simulink model "Test_Arithmetic_Operation_Word_Comparator_Equal"  (Simulink 8.7)
settings: Solver=ode45  StartTime=0.0  StopTime=len  RelTol=1e-3
libraries: Miscellaneous x2, Arithmetic_Operations_Lib x1
settings Model: Creator=uzivatel  LastModifiedBy=Jozko Mrkvicka
settings DebuggingCC: SolverPrmCheckMsg=warning  StateNameClashWarn=warning

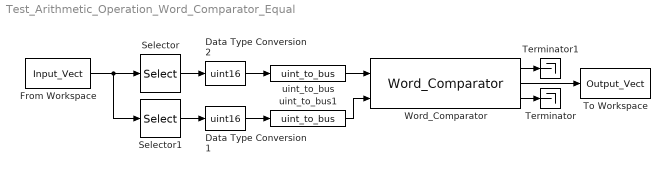
== system Test_Arithmetic_Operation_Word_Comparator_Equal ==
  Data Type Conversion1 : DataTypeConversion  OutDataTypeStr=uint16
  Data Type Conversion2 : DataTypeConversion  OutDataTypeStr=uint16
  From Workspace : FromWorkspace  VariableName=Input_Vect  SampleTime=1  Interpolate=off  OutputAfterFinalValue=Holding final value
  Selector : Selector  IndexMode=Zero-based  InputPortWidth=2  SampleTime=1  IndexOptions=Index vector (dialog)  Indices=0  OutputSizes=1
  Selector1 : Selector  IndexMode=Zero-based  InputPortWidth=2  SampleTime=1  IndexOptions=Index vector (dialog)  Indices=1  OutputSizes=1
  Terminator : Terminator
  Terminator1 : Terminator
  To Workspace : ToWorkspace  VariableName=Output_Vect  SampleTime=1
  Word_Comparator : Arithmetic_Operations_Lib/Arithmetic_Operations_Lib/Word_Comparator
  uint_to_bus : Miscellaneous/uint_to_bus
  uint_to_bus1 : Miscellaneous/uint_to_bus
  wires:
  From Workspace/1 -> Selector1/1, Selector/1
  Selector1/1 -> Data Type Conversion1/1
  Selector/1 -> Data Type Conversion2/1
  Data Type Conversion2/1 -> uint_to_bus/1
  Word_Comparator/3 -> Terminator/1
  Word_Comparator/2 -> To Workspace/1
  Data Type Conversion1/1 -> uint_to_bus1/1
  uint_to_bus/1 -> Word_Comparator/1
  uint_to_bus1/1 -> Word_Comparator/2
  Word_Comparator/1 -> Terminator1/1
